simulink model "PT2"  (R2020b)
settings: Solver=ode45  StartTime=0.0  StopTime=10.0  MaxStep=0.01  RelTol=1e-3
values from neighbouring files (symbols this model uses):
  K = 2    [init_PT2.m]
  T = 0.1    [init_PT2.m]
  y_0 = 1    [init_PT2.m]
  y_dot_0 = 0    [init_PT2.m]
  zeta = 0.2    [init_PT2.m]
settings Model: Creator=60251  LastModifiedBy=60251

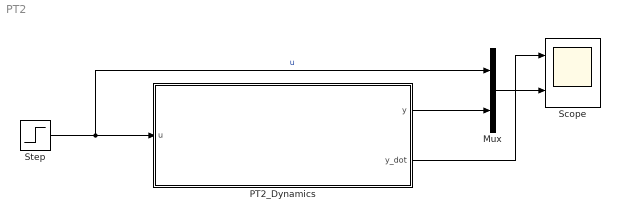
== system PT2 ==
  Mux : Mux  Inputs=2
  PT2_Dynamics : Subsystem
  Scope : Scope  NumInputPorts=2
  Step : Step  Time=5  SampleTime=0
  wires:
  Step/1 -> Mux/1, PT2_Dynamics/1(u)  "u"
  Mux/1 -> Scope/2
  PT2_Dynamics/2(y_dot) -> Scope/1
  PT2_Dynamics/1(y) -> Mux/2

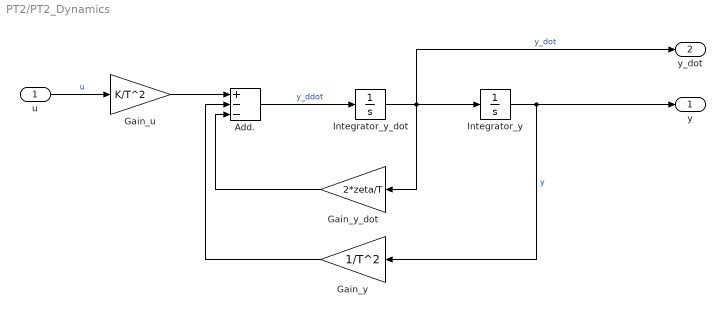
== system PT2/PT2_Dynamics ==
  u : Inport
  Add. : Sum  Inputs=+--
  Gain_u : Gain  Gain=K/T^2
  Gain_y : Gain  Gain=1/T^2
  Gain_y_dot : Gain  Gain=2*zeta/T
  Integrator_y : Integrator  InitialCondition=y_0
  Integrator_y_dot : Integrator  InitialCondition=y_dot_0
  y : Outport
  y_dot : Outport  Port=2
  wires:
  Gain_y_dot/1 -> Add./3
  u/1 -> Gain_u/1  "u"
  Gain_y/1 -> Add./2
  Integrator_y/1 -> y/1, Gain_y/1  "y"
  Add./1 -> Integrator_y_dot/1  "y_ddot"
  Integrator_y_dot/1 -> y_dot/1, Gain_y_dot/1, Integrator_y/1  "y_dot"
  Gain_u/1 -> Add./1
